simulink model "brain"  (Simulink 7.5)
settings: Solver=FixedStepDiscrete  StartTime=0.0  StopTime=inf  FixedStep=0.2  RelTol=1e-3
values from neighbouring files (symbols this model uses):
  Buoy1_Hue = 0.4    [brainconstants.m]    (also in brainconstants_David.m = 30)
  Buoy1_Saturation = 1.0    (= 1)    [brainconstants.m]    (also in brainconstants_David.m)
  Buoy1_Value = 0.45    [brainconstants.m]    (also in brainconstants_David.m)
  Buoy2_Hue = 0.0    (= 0)    [brainconstants.m]    (also in brainconstants_David.m = 80)
  Buoy2_Saturation = 1.0    (= 1)    [brainconstants.m]    (also in brainconstants_David.m)
  Buoy2_Value = 0.75    [brainconstants.m]    (also in brainconstants_David.m)
  Buoy_Max_Eccentricity = 0.7    [brainconstants.m]    (also in brainconstants_David.m = 1.2)
  Buoy_Max_Extent = 0.9    [brainconstants.m]    (also in brainconstants_David.m)
  Buoy_Min_Eccentricity = 0    [brainconstants.m]    (also in brainconstants_David.m)
  Buoy_Min_Extent = 0.7    [brainconstants.m]    (also in brainconstants_David.m = 0.1)
  Buoy_Strafe = 40    [brainconstants.m]    (also in brainconstants_David.m)
  Cam_Down_Strafe_XPos_Kd = 0.0    (= 0)    [brainconstants.m]    (also in brainconstants_David.m)
  Cam_Down_Strafe_XPos_Ki = 0.0    (= 0)    [brainconstants.m]    (also in brainconstants_David.m)
  Cam_Down_Strafe_XPos_Kp = -1.0    (= -1)    [brainconstants.m]    (also in brainconstants_David.m)
  Cam_Down_Yaw_XPos_Kd = 0.0    (= 0)    [brainconstants.m]    (also in brainconstants_David.m)
  Cam_Down_Yaw_XPos_Ki = 0.0    (= 0)    [brainconstants.m]    (also in brainconstants_David.m)
  Cam_Down_Yaw_XPos_Kp = 0.6    [brainconstants.m]    (also in brainconstants_David.m)
  Cam_Down_YPos_Kd = 0.0    (= 0)    [brainconstants.m]    (also in brainconstants_David.m)
  Cam_Down_YPos_Ki = 0.0    (= 0)    [brainconstants.m]    (also in brainconstants_David.m)
  Cam_Down_YPos_Kp = 0.75    [brainconstants.m]    (also in brainconstants_David.m)
  Cam_Forward_XPosition_Kd = 0.0    (= 0)    [brainconstants.m]    (also in brainconstants_David.m)
  Cam_Forward_XPosition_Ki = 0.0    (= 0)    [brainconstants.m]    (also in brainconstants_David.m)
  Cam_Forward_XPosition_Kp = 0.07    [brainconstants.m]    (also in brainconstants_David.m)
  Cam_Forward_YPosition_Kd = 0.0    (= 0)    [brainconstants.m]    (also in brainconstants_David.m)
  Cam_Forward_YPosition_Ki = 0.0    (= 0)    [brainconstants.m]    (also in brainconstants_David.m)
  Cam_Forward_YPosition_Kp = 0.8    [brainconstants.m]    (also in brainconstants_David.m)
  Depth_Kd = 0.0    (= 0)    [brainconstants.m]    (also in brainconstants_David.m)
  Depth_Ki = 0.0    (= 0)    [brainconstants.m]    (also in brainconstants_David.m)
  Depth_Kp = 75    [brainconstants.m]    (also in brainconstants_David.m)
  Heading_Forward_Velocity = 30    [brainconstants.m]    (also in brainconstants_David.m)
  Heading_Kd = 0.4    [brainconstants.m]    (also in brainconstants_David.m)
  Heading_Ki = 0.0    (= 0)    [brainconstants.m]    (also in brainconstants_David.m)
  Heading_Kp = 0.65    [brainconstants.m]    (also in brainconstants_David.m)
  Hedge_Hue = .4    (= 0.4)    [brainconstants.m]    (also in brainconstants_David.m)
  Hedge_Saturation = 1    [brainconstants.m]    (also in brainconstants_David.m)
  Hedge_Value = .75    (= 0.75)    [brainconstants.m]    (also in brainconstants_David.m)
  IMU_YawRate_Kd = 0.0    (= 0)    [brainconstants.m]    (also in brainconstants_David.m)
  IMU_YawRate_Ki = 0.0    (= 0)    [brainconstants.m]    (also in brainconstants_David.m)
  IMU_YawRate_Kp = 0.25    [brainconstants.m]    (also in brainconstants_David.m)
  IMU_YVel_Kd = 0.0    (= 0)    [brainconstants.m]    (also in brainconstants_David.m)
  IMU_YVel_Ki = 0.0    (= 0)    [brainconstants.m]    (also in brainconstants_David.m)
  IMU_YVel_Kp = 0.25    [brainconstants.m]    (also in brainconstants_David.m)
  Iter_Segment_Thresh = 60    [brainconstants.m]    (also in brainconstants_David.m)
  MissionPlan = [1 1 1 1 1 1 1 1 1 1 1 1 1 0 0 0 0 0 0 0]    [brainconstants.m]    (also in brainconstants_David.m)
  Track_Desired_Depth = 8    [brainconstants.m]    (also in brainconstants_David.m)
  Track_HueHigher = 0.75    [brainconstants.m]    (also in brainconstants_David.m)
  Track_HueLower = 0.4    [brainconstants.m]    (also in brainconstants_David.m)
  Track_Min_Eccentricity = 0.9    [brainconstants.m]    (also in brainconstants_David.m)
  Track_Saturation = 0.75    [brainconstants.m]    (also in brainconstants_David.m)
  Vision_Forward_Velocity = 15    [brainconstants.m]    (also in brainconstants_David.m)
undefined symbols (not defined in the file or in its folder): DiscIntNeverNeededParam, gray, Rec, SDTV, strel
libraries: vipconversions x32, simulink x26, vipgeotforms x9, vipstatistics x9, viptextngfix x7, vipmorphops x6, viptransforms x4, vipsnks x3, vipsrcs x1
(part 2 of 6)

== system brain/StateFlow Functions/StateFlowFunctions.GetDesiredDepth ==
  f : TriggerPort  TriggerType=function-call
      settings: CopyFcn=set_param(gcbh,'PreDeleteFcn','')  PreDeleteFcn=Stateflow.SLINSF.SimulinkMan.unsafePredeleteFcn
  Constant : Constant  Value=Track_Desired_Depth  OutDataType=fixdt(1, 16)  OutScaling=2^0  SampleTime=-1
  DesiredDepth : Outport
  wires:
  Constant/1 -> DesiredDepth/1

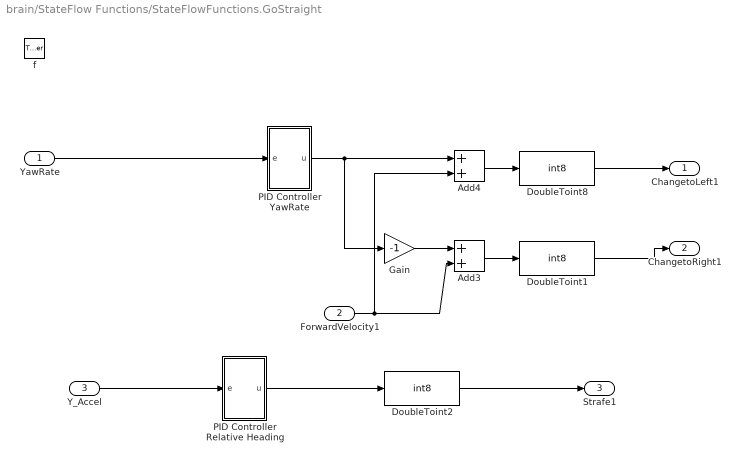
== system brain/StateFlow Functions/StateFlowFunctions.GoStraight ==
  YawRate : Inport
  ForwardVelocity1 : Inport  Port=2  OutDataType=fixdt(1, 16)  OutScaling=2^0
  Y_Accel : Inport  Port=3
  f : TriggerPort  TriggerType=function-call
      settings: CopyFcn=set_param(gcbh,'PreDeleteFcn','')  PreDeleteFcn=Stateflow.SLINSF.SimulinkMan.unsafePredeleteFcn
  Add3 : Sum  OutDataType=fixdt(1, 16)  OutScaling=2^-10
  Add4 : Sum  OutDataType=fixdt(1, 16)  OutScaling=2^-10
  DoubleToint1 : DataTypeConversion  OutDataTypeMode=int8  OutDataType=fixdt(1, 16)  OutScaling=2^0  OutDataTypeStr=int8  SaturateOnIntegerOverflow=on
  DoubleToint2 : DataTypeConversion  OutDataTypeMode=int8  OutDataType=fixdt(1, 16)  OutScaling=2^0  OutDataTypeStr=int8  SaturateOnIntegerOverflow=on
  DoubleToint8 : DataTypeConversion  OutDataTypeMode=int8  OutDataType=fixdt(1, 16)  OutScaling=2^0  OutDataTypeStr=int8  SaturateOnIntegerOverflow=on
  Gain : Gain  Gain=-1  ParameterDataType=fixdt(1, 16)  ParameterScaling=2^0  OutDataType=fixdt(1, 16)  OutScaling=2^0
  PID Controller Relative Heading : Subsystem  Description=PID
  PID Controller YawRate : Subsystem  Description=PID
  ChangetoLeft1 : Outport  OutDataType=fixdt(1, 16)  OutScaling=2^0
  ChangetoRight1 : Outport  Port=2  OutDataType=fixdt(1, 16)  OutScaling=2^0
  Strafe1 : Outport  Port=3  OutDataType=fixdt(1, 16)  OutScaling=2^0
  wires:
  PID Controller YawRate/1(u) -> Add4/1, Gain/1
  Add4/1 -> DoubleToint8/1
  Add3/1 -> DoubleToint1/1
  ForwardVelocity1/1 -> Add4/2, Add3/2
  YawRate/1 -> PID Controller YawRate/1(e)
  Gain/1 -> Add3/1
  DoubleToint8/1 -> ChangetoLeft1/1
  DoubleToint1/1 -> ChangetoRight1/1
  Y_Accel/1 -> PID Controller Relative Heading/1(e)
  PID Controller Relative Heading/1(u) -> DoubleToint2/1
  DoubleToint2/1 -> Strafe1/1

== system brain/StateFlow Functions/StateFlowFunctions.JumpHedge.ApproachHedge.GetArea ==
  BW : Inport  PortDimensions=[120 160]
  f : TriggerPort  TriggerType=function-call
      settings: CopyFcn=set_param(gcbh,'PreDeleteFcn','')  PreDeleteFcn=Stateflow.SLINSF.SimulinkMan.unsafePredeleteFcn
  Buoy Blob Analysis : vipstatistics/Blob Analysis  Tag=vipblks_row_conv  DialogController=vipDDGCreate  DialogControllerArgs=DataTag25  area=on  centroid=off  bBox=off  majorAxis=off  minorAxis=off  angle=off  eccentricity=off  equivDiameterSq=off  extent=off  perimeter=off  maxBlobs=Max_Num_Blobs  warnIfNumBlobsExceeded=off  isCount=off  useMinArea=on  minArea=Min_Blob_Size  useMaxArea=on  maxArea=Max_Blob_Size  excludeBorderBlob=off  outDT=double  isOutVarDim=off  isFill=on  fillValues=-1  conn=8  isLabel=off  outputMode=Binary point scaling  outputWordLength=32  outputFracLength=16  firstCoeffMode=Binary point scaling  firstCoeffWordLength=16  firstCoeffFracLength=14  secondCoeffMode=Binary point scaling  secondCoeffWordLength=32  secondCoeffFracLength=16  accumMode=Binary point scaling  accumWordLength=32  accumFracLength=0  prodOutputMode=Binary point scaling  prodOutputWordLength=32  prodOutputFracLength=16  roundingMode=Floor  overflowMode=off
  Dilation : vipmorphops/Dilation  nhoodsrc=Specify via dialog  strel=[1 1; 1 1]
  Embedded MATLAB Function : Stateflow chart  TreatAsAtomicUnit=on
  Erosion : vipmorphops/Erosion  nhoodsrc=Specify via dialog  strel=strel('square',4)
  Image Data Type Conversion : vipconversions/Image Data Type Conversion  outDT=boolean  isSigned=on  wordLen=16  numFracBits=0
  AreaBiggestBlob : Outport  OutDataType=fixdt(1, 16)  OutScaling=2^0
  wires:
  Buoy Blob Analysis/1 -> Embedded MATLAB Function/1(Area1)
  BW/1 -> Image Data Type Conversion/1  "BW"
  Dilation/1 -> Erosion/1
  Erosion/1 -> Buoy Blob Analysis/1, Embedded MATLAB Function/2(Image)
  Embedded MATLAB Function/1(BlobArea) -> AreaBiggestBlob/1
  Image Data Type Conversion/1 -> Dilation/1

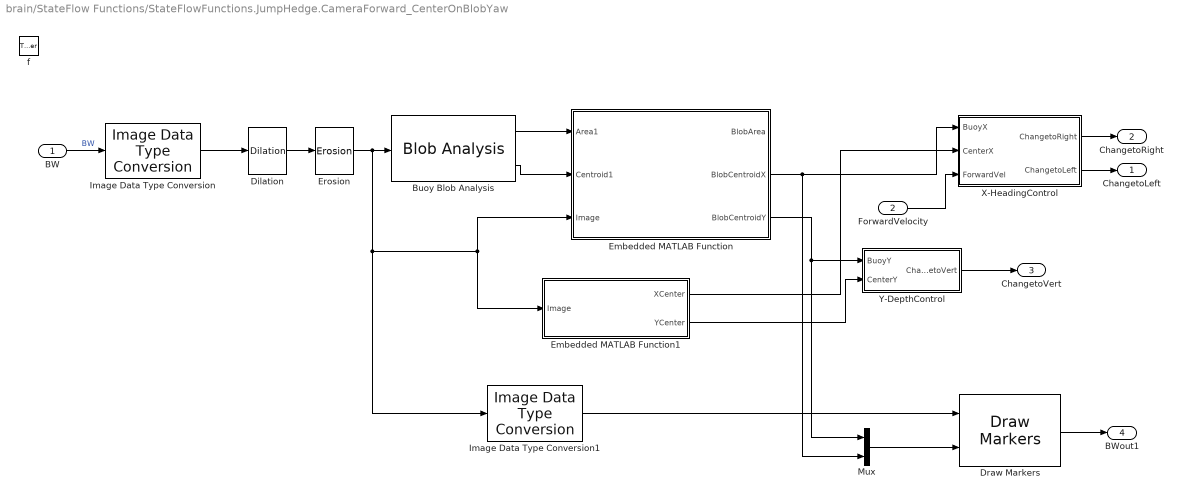
== system brain/StateFlow Functions/StateFlowFunctions.JumpHedge.CameraForward_CenterOnBlobYaw ==
  BW : Inport  PortDimensions=[120 160]
  ForwardVelocity : Inport  Port=2  PortDimensions=1
  f : TriggerPort  TriggerType=function-call
      settings: CopyFcn=set_param(gcbh,'PreDeleteFcn','')  PreDeleteFcn=Stateflow.SLINSF.SimulinkMan.unsafePredeleteFcn
  Buoy Blob Analysis : vipstatistics/Blob Analysis  Tag=vipblks_row_conv  DialogController=vipDDGCreate  DialogControllerArgs=DataTag26  area=on  centroid=on  bBox=off  majorAxis=off  minorAxis=off  angle=off  eccentricity=off  equivDiameterSq=off  extent=off  perimeter=off  maxBlobs=Max_Num_Blobs_Buoy  warnIfNumBlobsExceeded=off  isCount=off  useMinArea=on  minArea=Min_Blob_Size  useMaxArea=on  maxArea=Max_Blob_Size  excludeBorderBlob=off  outDT=double  isOutVarDim=off  isFill=on  fillValues=-1  conn=8  isLabel=off  outputMode=Binary point scaling  outputWordLength=32  outputFracLength=16  firstCoeffMode=Binary point scaling  firstCoeffWordLength=16  firstCoeffFracLength=14  secondCoeffMode=Binary point scaling  secondCoeffWordLength=32  secondCoeffFracLength=16  accumMode=Binary point scaling  accumWordLength=32  accumFracLength=0  prodOutputMode=Binary point scaling  prodOutputWordLength=32  prodOutputFracLength=16  roundingMode=Floor  overflowMode=off
  Dilation : vipmorphops/Dilation  nhoodsrc=Specify via dialog  strel=[1 1; 1 1]
  Draw Markers : viptextngfix/Draw Markers  DialogController=vipDDGCreate  DialogControllerArgs=DataTag27  shape=X-mark  size=7  fill=off  fillClrSource=Specify via dialog  display=User-specified value  intensity=200  color=.5  opacity=0.6  viewport=Entire image  antialiasing=off  inType=Obsolete  imagePorts=One multidimensional signal  prodOutputMode=Binary point scaling  prodOutputWordLength=32  prodOutputFracLength=14  memoryMode=Specify word length  memoryWordLength=16  memoryFracLength=15  roundingMode=Floor  overflowMode=off
  Embedded MATLAB Function : Stateflow chart  TreatAsAtomicUnit=on
  Embedded MATLAB Function1 : Stateflow chart  TreatAsAtomicUnit=on
  Erosion : vipmorphops/Erosion  nhoodsrc=Specify via dialog  strel=strel('square',4)
  Image Data Type Conversion : vipconversions/Image Data Type Conversion  outDT=boolean  isSigned=on  wordLen=16  numFracBits=0
  Image Data Type Conversion1 : vipconversions/Image Data Type Conversion  outDT=double  isSigned=on  wordLen=16  numFracBits=0
  Mux : Mux  Inputs=2
  X-HeadingControl : Subsystem
  Y-DepthControl : Subsystem
  ChangetoLeft : Outport  PortDimensions=1  OutDataType=fixdt(1, 16)  OutScaling=2^0
  ChangetoRight : Outport  Port=2  PortDimensions=1  OutDataType=fixdt(1, 16)  OutScaling=2^0
  ChangetoVert : Outport  Port=3  PortDimensions=1  OutDataType=fixdt(1, 16)  OutScaling=2^0
  BWout1 : Outport  Port=4  OutDataType=fixdt(1, 16)  OutScaling=2^0
  wires:
  X-HeadingControl/1(ChangetoRight) -> ChangetoRight/1
  X-HeadingControl/2(ChangetoLeft) -> ChangetoLeft/1
  Y-DepthControl/1(ChangetoVert) -> ChangetoVert/1
  Buoy Blob Analysis/1 -> Embedded MATLAB Function/1(Area1)
  Buoy Blob Analysis/2 -> Embedded MATLAB Function/2(Centroid1)
  Embedded MATLAB Function/2(BlobCentroidX) -> X-HeadingControl/1(BuoyX), Mux/2
  Embedded MATLAB Function/3(BlobCentroidY) -> Y-DepthControl/1(BuoyY), Mux/1
  BW/1 -> Image Data Type Conversion/1  "BW"
  Embedded MATLAB Function1/1(XCenter) -> X-HeadingControl/2(CenterX)
  Embedded MATLAB Function1/2(YCenter) -> Y-DepthControl/2(CenterY)
  Dilation/1 -> Erosion/1
  Erosion/1 -> Buoy Blob Analysis/1, Embedded MATLAB Function/3(Image), Embedded MATLAB Function1/1(Image), Image Data Type Conversion1/1
  ForwardVelocity/1 -> X-HeadingControl/3(ForwardVel)
  Image Data Type Conversion/1 -> Dilation/1
  Mux/1 -> Draw Markers/2
  Image Data Type Conversion1/1 -> Draw Markers/1
  Draw Markers/1 -> BWout1/1

== system brain/StateFlow Functions/StateFlowFunctions.JumpHedge.GetAxisRatio ==
  BW : Inport  PortDimensions=[120 160]
  f : TriggerPort  TriggerType=function-call
      settings: CopyFcn=set_param(gcbh,'PreDeleteFcn','')  PreDeleteFcn=Stateflow.SLINSF.SimulinkMan.unsafePredeleteFcn
  Blob Analysis : vipstatistics/Blob Analysis  Tag=vipblks_row_conv  DialogController=vipDDGCreate  DialogControllerArgs=DataTag28  area=on  centroid=off  bBox=on  majorAxis=off  minorAxis=off  angle=off  eccentricity=off  equivDiameterSq=off  extent=off  perimeter=off  maxBlobs=10  warnIfNumBlobsExceeded=on  isCount=off  useMinArea=off  minArea=0  useMaxArea=off  maxArea=intmax('uint32')  excludeBorderBlob=off  outDT=double  isOutVarDim=off  isFill=on  fillValues=-1  conn=8  isLabel=off  outputMode=Binary point scaling  outputWordLength=32  outputFracLength=16  firstCoeffMode=Binary point scaling  firstCoeffWordLength=16  firstCoeffFracLength=14  secondCoeffMode=Binary point scaling  secondCoeffWordLength=32  secondCoeffFracLength=16  accumMode=Binary point scaling  accumWordLength=32  accumFracLength=0  prodOutputMode=Binary point scaling  prodOutputWordLength=32  prodOutputFracLength=16  roundingMode=Floor  overflowMode=off
  Embedded MATLAB Function : Stateflow chart  TreatAsAtomicUnit=on
  Image Data Type Conversion : vipconversions/Image Data Type Conversion  outDT=boolean  isSigned=on  wordLen=16  numFracBits=0
  AxisRatio : Outport
  wires:
  BW/1 -> Image Data Type Conversion/1
  Blob Analysis/1 -> Embedded MATLAB Function/1(Area1)
  Blob Analysis/2 -> Embedded MATLAB Function/2(BBox)
  Embedded MATLAB Function/2(AxisRatio) -> AxisRatio/1
  Image Data Type Conversion/1 -> Blob Analysis/1, Embedded MATLAB Function/3(Image)

== system brain/StateFlow Functions/StateFlowFunctions.JumpHedge.GetForwardVelocity ==
  f : TriggerPort  TriggerType=function-call
      settings: CopyFcn=set_param(gcbh,'PreDeleteFcn','')  PreDeleteFcn=Stateflow.SLINSF.SimulinkMan.unsafePredeleteFcn
  Heading Forward Velocity : Constant  Value=Vision_Forward_Velocity  OutDataType=fixdt(1, 16)  OutScaling=2^0  SampleTime=-1
  ForwardVel : Outport
  wires:
  Heading Forward Velocity/1 -> ForwardVel/1

== system brain/StateFlow Functions/StateFlowFunctions.JumpHedge.IndividualSegmentation ==
  LabMatrix : Inport  PortDimensions=[120 160]
  Ref_Colors : Inport  Port=2  PortDimensions=[50 3]
  Num_Colors : Inport  Port=3  PortDimensions=1
  B_Hue : Inport  Port=4
  B_Sat : Inport  Port=5
  B_Value : Inport  Port=6
  f : TriggerPort  TriggerType=function-call
      settings: CopyFcn=set_param(gcbh,'PreDeleteFcn','')  PreDeleteFcn=Stateflow.SLINSF.SimulinkMan.unsafePredeleteFcn
  Threshold The Image : Subsystem
  BW : Outport  PortDimensions=[120 160]  OutDataType=fixdt(1, 16)  OutScaling=2^0
  wires:
  LabMatrix/1 -> Threshold The Image/1(LabelMatrix)
  Ref_Colors/1 -> Threshold The Image/2(ref_colors)
  Num_Colors/1 -> Threshold The Image/3(num_colors)
  B_Hue/1 -> Threshold The Image/4(H_Hue)
  B_Sat/1 -> Threshold The Image/5(H_Sat)
  B_Value/1 -> Threshold The Image/6(H_Value)
  Threshold The Image/1(BW) -> BW/1

== system brain/StateFlow Functions/StateFlowFunctions.JumpHedge.IterativeSegmentation ==
  H : Inport  PortDimensions=[120 160]
  S : Inport  Port=2  PortDimensions=[120 160]
  V : Inport  Port=3  PortDimensions=[120 160]
  f : TriggerPort  TriggerType=function-call
      settings: CopyFcn=set_param(gcbh,'PreDeleteFcn','')  PreDeleteFcn=Stateflow.SLINSF.SimulinkMan.unsafePredeleteFcn
  Color Space  Conversion : vipconversions/Color Space  Conversion  conversion=Obsolete  conversionActive=HSV to R'G'B'  wp_str=D50  rec=Rec. 601 (SDTV)  sys=1125/60/2:1  imagePorts=Separate color signals
  Color Space  Conversion1 : vipconversions/Color Space  Conversion  conversion=Obsolete  conversionActive=sR'G'B' to L*a*b*  wp_str=D50  rec=Rec. 601 (SDTV)  sys=1125/60/2:1  imagePorts=Separate color signals
  Low Pass Filter : Subsystem
  Segmentation : Subsystem
  LabelMatrix : Outport  PortDimensions=[120 160]
  num_colors : Outport  Port=2
  Ref_Colors : Outport  Port=3
  wires:
  Color Space  Conversion/1 -> Low Pass Filter/1(R)
  Color Space  Conversion/2 -> Low Pass Filter/2(G)
  Color Space  Conversion/3 -> Low Pass Filter/3(B)
  Color Space  Conversion1/1 -> Segmentation/1(L)
  Color Space  Conversion1/2 -> Segmentation/2(a)
  Color Space  Conversion1/3 -> Segmentation/3(b)
  Low Pass Filter/1(R') -> Color Space  Conversion1/1
  Low Pass Filter/2(G') -> Color Space  Conversion1/2
  Low Pass Filter/3(B') -> Color Space  Conversion1/3
  H/1 -> Color Space  Conversion/1
  S/1 -> Color Space  Conversion/2
  V/1 -> Color Space  Conversion/3
  Segmentation/1(LabelMatrix) -> LabelMatrix/1
  Segmentation/2(num_colors) -> num_colors/1
  Segmentation/3(ref_colors) -> Ref_Colors/1

== system brain/StateFlow Functions/StateFlowFunctions.JumpHedge.RecognizeHedge.GetHedgeValues ==
  f : TriggerPort  TriggerType=function-call
      settings: CopyFcn=set_param(gcbh,'PreDeleteFcn','')  PreDeleteFcn=Stateflow.SLINSF.SimulinkMan.unsafePredeleteFcn
  Hedge Hue : Constant  Value=Hedge_Hue  OutDataType=fixdt(1, 16)  OutScaling=2^0  SampleTime=-1
  Hedge Saturation : Constant  Value=Hedge_Saturation  OutDataType=fixdt(1, 16)  OutScaling=2^0  SampleTime=-1
  Hedge Value : Constant  Value=Hedge_Value  OutDataType=fixdt(1, 16)  OutScaling=2^0  SampleTime=-1
  H_hue : Outport
  H_sat : Outport  Port=2
  H_val : Outport  Port=3
  wires:
  Hedge Hue/1 -> H_hue/1
  Hedge Saturation/1 -> H_sat/1
  Hedge Value/1 -> H_val/1

== system brain/StateFlow Functions/StateFlowFunctions.JumpHedge.RecognizeHedge.LookForHedge ==
  BW : Inport  PortDimensions=[120 160]
  f : TriggerPort  TriggerType=function-call
      settings: CopyFcn=set_param(gcbh,'PreDeleteFcn','')  PreDeleteFcn=Stateflow.SLINSF.SimulinkMan.unsafePredeleteFcn
  Are 3 Lines Present : Stateflow chart  TreatAsAtomicUnit=on
  Draw Shapes : viptextngfix/Draw Shapes  DialogController=vipDDGCreate  DialogControllerArgs=DataTag32  shape=Lines  fill=off  fillClrSource=Specify via dialog  display=User-specified value  intensity=200  color=.8  opacity=0.6  viewport=Entire image  antialiasing=off  inType=Obsolete  imagePorts=One multidimensional signal  prodOutputMode=Binary point scaling  prodOutputWordLength=32  prodOutputFracLength=14  memoryMode=Specify word length  memoryWordLength=16  memoryFracLength=15  roundingMode=Floor  overflowMode=off
  Erosion : vipmorphops/Erosion  nhoodsrc=Specify via dialog  strel=[1 1 1;1 1 1]
  Hough Lines : viptransforms/Hough Lines  DialogController=vipDDGCreate  DialogControllerArgs=DataTag33  sineCompMethod=Trigonometric function  thetaRes=pi/180  firstCoeffMode=Specify word length  firstCoeffWordLength=16  firstCoeffFracLength=15  prodOutputMode=Binary point scaling  prodOutputWordLength=32  prodOutputFracLength=16  roundingMode=Nearest  overflowMode=on
  Hough Transform : viptransforms/Hough Transform  DialogController=vipDDGCreate  DialogControllerArgs=DataTag34  theta_res=pi/180  rho_res=1  out_theta_rho=on  outdtmode=double  firstCoeffMode=Binary point scaling  firstCoeffWordLength=16  firstCoeffFracLength=14  secondCoeffMode=Binary point scaling  secondCoeffWordLength=32  secondCoeffFracLength=16  outputMode=Binary point scaling  outputWordLength=16  outputFracLength=0  accumMode=Binary point scaling  accumWordLength=32  accumFracLength=20  prodOutputMode=Binary point scaling  prodOutputWordLength=32  prodOutputFracLength=20  memoryMode=Binary point scaling  memoryWordLength=32  memoryFracLength=16  roundingMode=Nearest  overflowMode=on
  Image Data Type Conversion : vipconversions/Image Data Type Conversion  outDT=boolean  isSigned=on  wordLen=16  numFracBits=0
  Image1 : Outport
  BWout1 : Outport  Port=2  PortDimensions=[120 160]
  wires:
  BW/1 -> Image Data Type Conversion/1, Hough Lines/3, Draw Shapes/1
  Hough Transform/1 -> Are 3 Lines Present/1(HoughTable)
  Hough Transform/2 -> Are 3 Lines Present/2(Theta)
  Hough Transform/3 -> Are 3 Lines Present/3(Rho)
  Are 3 Lines Present/1(Image) -> Image1/1
  Are 3 Lines Present/2(T) -> Hough Lines/1
  Are 3 Lines Present/3(R) -> Hough Lines/2
  Hough Lines/1 -> Draw Shapes/2
  Draw Shapes/1 -> BWout1/1
  Erosion/1 -> Hough Transform/1
  Image Data Type Conversion/1 -> Erosion/1

== system brain/StateFlow Functions/StateFlowFunctions.JumpHedge.ShowSegmentedImage ==
  LabMatrix : Inport  PortDimensions=[120 160]
  Ref_Colors : Inport  Port=2  PortDimensions=[50 3]
  f : TriggerPort  TriggerType=function-call
      settings: CopyFcn=set_param(gcbh,'PreDeleteFcn','')  PreDeleteFcn=Stateflow.SLINSF.SimulinkMan.unsafePredeleteFcn
  Color Space  Conversion : vipconversions/Color Space  Conversion  conversion=Obsolete  conversionActive=L*a*b* to sR'G'B'  wp_str=D50  rec=Rec. 601 (SDTV)  sys=1125/60/2:1  imagePorts=Separate color signals
  Embedded MATLAB Function : Stateflow chart  TreatAsAtomicUnit=on
  Embedded MATLAB Function1 : Stateflow chart  TreatAsAtomicUnit=on
  RGBout : Outport  PortDimensions=[120 160 3]  OutDataType=fixdt(1, 16)  OutScaling=2^0
  wires:
  LabMatrix/1 -> Embedded MATLAB Function/1(LabMatrix)
  Ref_Colors/1 -> Embedded MATLAB Function/2(Ref_Colors)
  Embedded MATLAB Function/1(L) -> Color Space  Conversion/1
  Embedded MATLAB Function/2(a) -> Color Space  Conversion/2
  Embedded MATLAB Function/3(b) -> Color Space  Conversion/3
  Color Space  Conversion/1 -> Embedded MATLAB Function1/1(R)
  Color Space  Conversion/2 -> Embedded MATLAB Function1/2(G)
  Color Space  Conversion/3 -> Embedded MATLAB Function1/3(B)
  Embedded MATLAB Function1/1(RGB) -> RGBout/1

== system brain/StateFlow Functions/StateFlowFunctions.LocatePinger.GetPingerHeading.GetHeadings ==
  f : TriggerPort  TriggerType=function-call
      settings: CopyFcn=set_param(gcbh,'PreDeleteFcn','')  PreDeleteFcn=Stateflow.SLINSF.SimulinkMan.unsafePredeleteFcn
  Heading11 : Outport
  Heading22 : Outport  Port=2

== system brain/StateFlow Functions/StateFlowFunctions.MaintainDepth ==
  note: Error
  CurrentDepth1 : Inport  DataType=single  OutDataType=fixdt(1, 16)  OutScaling=2^0  OutDataTypeStr=single
  DesiredDepth1 : Inport  Port=2  DataType=single  OutDataType=fixdt(1, 16)  OutScaling=2^0  OutDataTypeStr=single
  f : TriggerPort  TriggerType=function-call
      settings: CopyFcn=set_param(gcbh,'PreDeleteFcn','')  PreDeleteFcn=Stateflow.SLINSF.SimulinkMan.unsafePredeleteFcn
  Add : Sum  Inputs=+-  OutDataTypeMode=double  OutDataType=fixdt(1, 16)  OutScaling=2^-10  OutDataTypeStr=double
  Double To Int8 : DataTypeConversion  OutDataTypeMode=int8  OutDataType=fixdt(1, 16)  OutScaling=2^0  OutDataTypeStr=int8  SaturateOnIntegerOverflow=on
  PID Controller Depth S3 : Subsystem  Description=PID
  ChangetoVertical : Outport  DataType=int8  OutDataType=fixdt(1, 16)  OutScaling=2^0  OutDataTypeStr=int8
  wires:
  DesiredDepth1/1 -> Add/1
  CurrentDepth1/1 -> Add/2
  Double To Int8/1 -> ChangetoVertical/1
  PID Controller Depth S3/1(u) -> Double To Int8/1
  Add/1 -> PID Controller Depth S3/1(e)

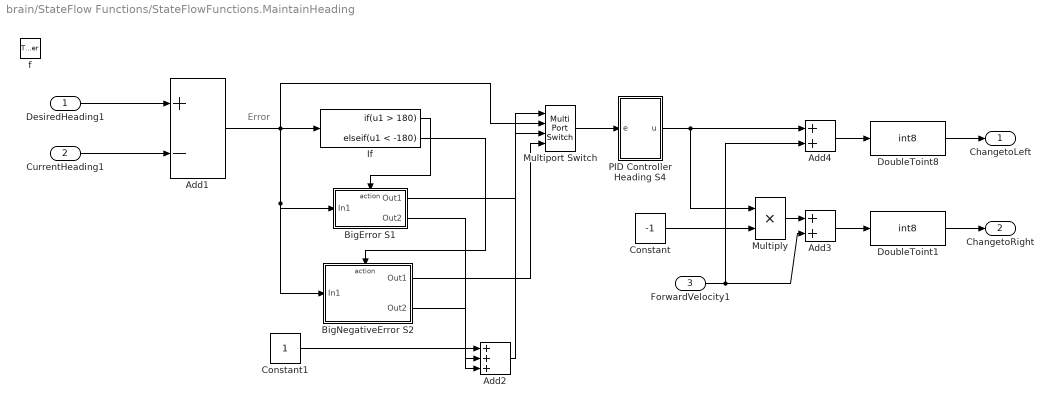
== system brain/StateFlow Functions/StateFlowFunctions.MaintainHeading ==
  note: Error
  DesiredHeading1 : Inport  PortDimensions=1  OutDataType=fixdt(1, 16)  OutScaling=2^0
  CurrentHeading1 : Inport  Port=2  PortDimensions=1  OutDataType=fixdt(1, 16)  OutScaling=2^0
  ForwardVelocity1 : Inport  Port=3  OutDataType=fixdt(1, 16)  OutScaling=2^0
  f : TriggerPort  TriggerType=function-call
      settings: CopyFcn=set_param(gcbh,'PreDeleteFcn','')  PreDeleteFcn=Stateflow.SLINSF.SimulinkMan.unsafePredeleteFcn
  Add1 : Sum  Inputs=+-  AccumDataTypeStr=double  OutDataType=fixdt(1, 16)  OutScaling=2^-10
  Add2 : Sum  Inputs=+++  OutDataType=fixdt(1, 16)  OutScaling=2^-10
  Add3 : Sum  OutDataType=fixdt(1, 16)  OutScaling=2^-10
  Add4 : Sum  OutDataType=fixdt(1, 16)  OutScaling=2^-10
  BigError S1 : Subsystem  TreatAsAtomicUnit=on
  BigNegativeError S2 : Subsystem  TreatAsAtomicUnit=on
  Constant : Constant  Value=-1  OutDataTypeMode=int8  OutDataType=fixdt(1, 16)  OutScaling=2^0  OutDataTypeStr=int8  SampleTime=-1
  Constant1 : Constant  OutDataType=fixdt(1, 16)  OutScaling=2^0  SampleTime=-1
  DoubleToint1 : DataTypeConversion  OutDataTypeMode=int8  OutDataType=fixdt(1, 16)  OutScaling=2^0  OutDataTypeStr=int8  SaturateOnIntegerOverflow=on
  DoubleToint8 : DataTypeConversion  OutDataTypeMode=int8  OutDataType=fixdt(1, 16)  OutScaling=2^0  OutDataTypeStr=int8  SaturateOnIntegerOverflow=on
  If : If  IfExpression=u1 > 180  ElseIfExpressions=u1 < -180  ShowElse=off
  Multiply : Product  Inputs=**  OutDataTypeMode=int8  OutDataType=fixdt(1, 16)  OutScaling=2^-10  OutDataTypeStr=int8
  Multiport Switch : MultiPortSwitch  zeroidx=off  OutDataType=fixdt(1, 16)  OutScaling=2^0
  PID Controller Heading S4 : Subsystem  Description=PID
  ChangetoLeft : Outport  OutDataType=fixdt(1, 16)  OutScaling=2^0
  ChangetoRight : Outport  Port=2  OutDataType=fixdt(1, 16)  OutScaling=2^0
  wires:
  PID Controller Heading S4/1(u) -> Multiply/1, Add4/1
  DoubleToint8/1 -> ChangetoLeft/1
  Add4/1 -> DoubleToint8/1
  DoubleToint1/1 -> ChangetoRight/1
  Add3/1 -> DoubleToint1/1
  ForwardVelocity1/1 -> Add4/2, Add3/2
  Multiply/1 -> Add3/1
  CurrentHeading1/1 -> Add1/2
  Add2/1 -> Multiport Switch/1
  BigNegativeError S2/2(Out2) -> Add2/3
  BigError S1/2(Out2) -> Add2/2
  Constant1/1 -> Add2/1
  Multiport Switch/1 -> PID Controller Heading S4/1(e)
  BigNegativeError S2/1(Out1) -> Multiport Switch/4
  BigError S1/1(Out1) -> Multiport Switch/3
  If/2 -> BigNegativeError S2/Action
  If/1 -> BigError S1/Action
  Add1/1 -> Multiport Switch/2, If/1, BigNegativeError S2/1(In1), BigError S1/1(In1)
  Constant/1 -> Multiply/2
  DesiredHeading1/1 -> Add1/1

== system brain/StateFlow Functions/StateFlowFunctions.ValidationGate.GetValidationGateForwardVelocity ==
  f : TriggerPort  TriggerType=function-call
      settings: CopyFcn=set_param(gcbh,'PreDeleteFcn','')  PreDeleteFcn=Stateflow.SLINSF.SimulinkMan.unsafePredeleteFcn
  Heading Forward Velocity : Constant  Value=Heading_Forward_Velocity  OutDataType=fixdt(1, 16)  OutScaling=2^0  SampleTime=-1
  ForwardVel : Outport
  wires:
  Heading Forward Velocity/1 -> ForwardVel/1

== system brain/StateFlow Functions/StateFlowFunctions.ValidationGate.LookforTrack ==
  H : Inport  PortDimensions=[120 160]  OutDataType=fixdt(1, 16)  OutScaling=2^0
  S : Inport  Port=2  PortDimensions=[120 160]  OutDataType=fixdt(1, 16)  OutScaling=2^0
  f : TriggerPort  TriggerType=function-call
      settings: CopyFcn=set_param(gcbh,'PreDeleteFcn','')  PreDeleteFcn=Stateflow.SLINSF.SimulinkMan.unsafePredeleteFcn
  LookforTrack : Subsystem
  Image : Outport  OutDataType=fixdt(1, 16)  OutScaling=2^0
  BWout1 : Outport  Port=2  OutDataType=fixdt(1, 16)  OutScaling=2^0
  wires:
  H/1 -> LookforTrack/1(H)
  S/1 -> LookforTrack/2(S)
  LookforTrack/1(BWout) -> BWout1/1
  LookforTrack/2(Image) -> Image/1

== system brain/StateFlow Functions/StateManagement.Running.Autonomous.Perform ==
  State1 : Inport
  f : TriggerPort  TriggerType=function-call
      settings: CopyFcn=set_param(gcbh,'PreDeleteFcn','')  PreDeleteFcn=Stateflow.SLINSF.SimulinkMan.unsafePredeleteFcn
  Checking to see if state will be performed : Stateflow chart  TreatAsAtomicUnit=on
  Mission Plan : Constant  Value=MissionPlan  OutDataType=fixdt(1, 16)  OutScaling=2^0  SampleTime=-1
  Done1 : Outport
  wires:
  State1/1 -> Checking to see if state will be performed/1(State1)
  Mission Plan/1 -> Checking to see if state will be performed/2(MissionPlan)
  Checking to see if state will be performed/1(Done1) -> Done1/1

== system brain/StateFlow Functions/StateFlowFunctions.Buoys.ApproachBuoys.ApproachFirstBuoy.WhichBuoysToApproach/FirstBuoy Info ==
  Color Space  Conversion : vipconversions/Color Space  Conversion  conversion=Obsolete  conversionActive=HSV to R'G'B'  wp_str=D65  rec=Rec. 601 (SDTV)  sys=1125/60/2:1  imagePorts=Separate color signals
  Color Space  Conversion1 : vipconversions/Color Space  Conversion  conversion=Obsolete  conversionActive=sR'G'B' to L*a*b*  wp_str=D50  rec=Rec. 601 (SDTV)  sys=1125/60/2:1  imagePorts=Separate color signals
  Constant : Constant  Value=Buoy1_Hue  OutDataType=fixdt(1, 16)  OutScaling=2^0  SampleTime=-1
  Constant1 : Constant  Value=Buoy1_Value  OutDataType=fixdt(1, 16)  OutScaling=2^0  SampleTime=-1
  Constant2 : Constant  Value=Buoy1_Saturation  OutDataType=fixdt(1, 16)  OutScaling=2^0  SampleTime=-1
  Out1 : Outport
  Out2 : Outport  Port=2
  Out3 : Outport  Port=3
  wires:
  Color Space  Conversion/1 -> Color Space  Conversion1/1
  Color Space  Conversion/2 -> Color Space  Conversion1/2
  Color Space  Conversion/3 -> Color Space  Conversion1/3
  Constant/1 -> Color Space  Conversion/1
  Constant2/1 -> Color Space  Conversion/2
  Constant1/1 -> Color Space  Conversion/3
  Color Space  Conversion1/1 -> Out1/1
  Color Space  Conversion1/2 -> Out2/1
  Color Space  Conversion1/3 -> Out3/1

== system brain/StateFlow Functions/StateFlowFunctions.Buoys.ApproachBuoys.ApproachFirstBuoy.WhichBuoysToApproach/Second Buoy Info ==
  Color Space  Conversion : vipconversions/Color Space  Conversion  conversion=Obsolete  conversionActive=HSV to R'G'B'  wp_str=D65  rec=Rec. 601 (SDTV)  sys=1125/60/2:1  imagePorts=Separate color signals
  Color Space  Conversion1 : vipconversions/Color Space  Conversion  conversion=Obsolete  conversionActive=sR'G'B' to L*a*b*  wp_str=D50  rec=Rec. 601 (SDTV)  sys=1125/60/2:1  imagePorts=Separate color signals
  Constant : Constant  Value=Buoy2_Hue  OutDataType=fixdt(1, 16)  OutScaling=2^0  SampleTime=-1
  Constant1 : Constant  Value=Buoy2_Value  OutDataType=fixdt(1, 16)  OutScaling=2^0  SampleTime=-1
  Constant2 : Constant  Value=Buoy2_Saturation  OutDataType=fixdt(1, 16)  OutScaling=2^0  SampleTime=-1
  Out1 : Outport
  Out2 : Outport  Port=2
  Out3 : Outport  Port=3
  wires:
  Color Space  Conversion/1 -> Color Space  Conversion1/1
  Color Space  Conversion/2 -> Color Space  Conversion1/2
  Color Space  Conversion/3 -> Color Space  Conversion1/3
  Constant/1 -> Color Space  Conversion/1
  Constant2/1 -> Color Space  Conversion/2
  Constant1/1 -> Color Space  Conversion/3
  Color Space  Conversion1/1 -> Out1/1
  Color Space  Conversion1/2 -> Out2/1
  Color Space  Conversion1/3 -> Out3/1

== system brain/StateFlow Functions/StateFlowFunctions.Buoys.ApproachBuoys.Buoy/Threshold The Image ==
  LabelMatrix : Inport
  ref_colors : Inport  Port=2
  num_colors : Inport  Port=3
  B_Hue : Inport  Port=4
  B_Sat : Inport  Port=5
  B_Value : Inport  Port=6
  Choose Closest Color : Stateflow chart  TreatAsAtomicUnit=on
  Get Desired Color : Subsystem
  Relational Operator : RelationalOperator  Operator===  LogicOutDataTypeMode=boolean  LogicDataType=fixdt(0, 8)  OutDataTypeStr=boolean
  BW : Outport
  wires:
  Relational Operator/1 -> BW/1  "BW"
  ref_colors/1 -> Choose Closest Color/1(ref_colors)
  num_colors/1 -> Choose Closest Color/2(num_colors)
  Get Desired Color/1(L) -> Choose Closest Color/3(L)
  Get Desired Color/2(a) -> Choose Closest Color/4(a)
  Get Desired Color/3(b) -> Choose Closest Color/5(b)
  LabelMatrix/1 -> Relational Operator/1
  Choose Closest Color/1(index) -> Relational Operator/2
  B_Hue/1 -> Get Desired Color/1(B_Hue)
  B_Sat/1 -> Get Desired Color/2(B_Sat)
  B_Value/1 -> Get Desired Color/3(B_Value)

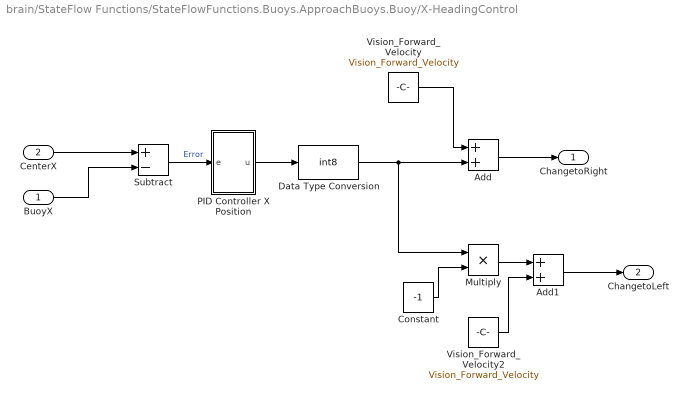
== system brain/StateFlow Functions/StateFlowFunctions.Buoys.ApproachBuoys.Buoy/X-HeadingControl ==
  BuoyX : Inport  OutDataType=fixdt(1, 16)  OutScaling=2^0
  CenterX : Inport  Port=2  OutDataType=fixdt(1, 16)  OutScaling=2^0
  Add : Sum  OutDataType=fixdt(1, 16)  OutScaling=2^-10
  Add1 : Sum  OutDataType=fixdt(1, 16)  OutScaling=2^-10
  Constant : Constant  Value=-1  OutDataType=fixdt(1, 16)  OutScaling=2^0  SampleTime=-1
  Data Type Conversion : DataTypeConversion  OutDataTypeMode=int8  OutDataType=fixdt(1, 16)  OutScaling=2^0  OutDataTypeStr=int8  SaturateOnIntegerOverflow=on
  Multiply : Product  Inputs=**  OutDataType=fixdt(1, 16)  OutScaling=2^-10
  PID Controller X Position : Subsystem  Description=PID
  Subtract : Sum  Inputs=+-  OutDataTypeMode=double  OutDataType=fixdt(1, 16)  OutScaling=2^-10  OutDataTypeStr=double
  Vision_Forward_Velocity : Constant  Value=Vision_Forward_Velocity  OutDataType=fixdt(1, 16)  OutScaling=2^0  SampleTime=-1
  Vision_Forward_Velocity2 : Constant  Value=Vision_Forward_Velocity  OutDataType=fixdt(1, 16)  OutScaling=2^0  SampleTime=-1
  ChangetoRight : Outport  OutDataType=fixdt(1, 16)  OutScaling=2^0
  ChangetoLeft : Outport  Port=2  OutDataType=fixdt(1, 16)  OutScaling=2^0
  wires:
  CenterX/1 -> Subtract/1
  BuoyX/1 -> Subtract/2
  Subtract/1 -> PID Controller X Position/1(e)  "Error"
  PID Controller X Position/1(u) -> Data Type Conversion/1
  Constant/1 -> Multiply/2
  Data Type Conversion/1 -> Multiply/1, Add/2
  Vision_Forward_Velocity/1 -> Add/1
  Add/1 -> ChangetoRight/1
  Multiply/1 -> Add1/1
  Vision_Forward_Velocity2/1 -> Add1/2
  Add1/1 -> ChangetoLeft/1

== system brain/StateFlow Functions/StateFlowFunctions.Buoys.ApproachBuoys.Buoy/Y-DepthControl ==
  BuoyY : Inport  OutDataType=fixdt(1, 16)  OutScaling=2^0
  CenterY : Inport  Port=2  OutDataType=fixdt(1, 16)  OutScaling=2^0
  Data Type Conversion : DataTypeConversion  OutDataTypeMode=int8  OutDataType=fixdt(1, 16)  OutScaling=2^0  OutDataTypeStr=int8  SaturateOnIntegerOverflow=on
  PID Controller Y Position : Subsystem  Description=PID
  Subtract : Sum  Inputs=-+  OutDataTypeMode=double  OutDataType=fixdt(1, 16)  OutScaling=2^-10  OutDataTypeStr=double
  ChangetoVert : Outport  OutDataType=fixdt(1, 16)  OutScaling=2^0
  wires:
  CenterY/1 -> Subtract/1
  BuoyY/1 -> Subtract/2
  Subtract/1 -> PID Controller Y Position/1(e)  "Error"
  PID Controller Y Position/1(u) -> Data Type Conversion/1
  Data Type Conversion/1 -> ChangetoVert/1

== system brain/StateFlow Functions/StateFlowFunctions.Buoys.ApproachBuoys.FindSecondBuoy.SecondBuoy/Threshold The Image ==
  LabelMatrix : Inport
  ref_colors : Inport  Port=2
  num_colors : Inport  Port=3
  B_Hue : Inport  Port=4
  B_Sat : Inport  Port=5
  B_Value : Inport  Port=6
  Choose Closest Color : Stateflow chart  TreatAsAtomicUnit=on
  Get Desired Color : Subsystem
  Relational Operator : RelationalOperator  Operator===  LogicOutDataTypeMode=boolean  LogicDataType=fixdt(0, 8)  OutDataTypeStr=boolean
  BW : Outport
  wires:
  Relational Operator/1 -> BW/1  "BW"
  ref_colors/1 -> Choose Closest Color/1(ref_colors)
  num_colors/1 -> Choose Closest Color/2(num_colors)
  Get Desired Color/1(L) -> Choose Closest Color/3(L)
  Get Desired Color/2(a) -> Choose Closest Color/4(a)
  Get Desired Color/3(b) -> Choose Closest Color/5(b)
  LabelMatrix/1 -> Relational Operator/1
  Choose Closest Color/1(index) -> Relational Operator/2
  B_Hue/1 -> Get Desired Color/1(B_Hue)
  B_Sat/1 -> Get Desired Color/2(B_Sat)
  B_Value/1 -> Get Desired Color/3(B_Value)

== system brain/StateFlow Functions/StateFlowFunctions.Buoys.IterativeSegmentation/Low Pass Filter ==
  R : Inport
  G : Inport  Port=2
  B : Inport  Port=3
  Low Pass Filter : Stateflow chart  TreatAsAtomicUnit=on
  Low Pass Filter1 : Stateflow chart  TreatAsAtomicUnit=on
  Low Pass Filter2 : Stateflow chart  TreatAsAtomicUnit=on
  R' : Outport
  G' : Outport  Port=2
  B' : Outport  Port=3
  wires:
  R/1 -> Low Pass Filter/1(I)
  G/1 -> Low Pass Filter1/1(I)
  B/1 -> Low Pass Filter2/1(I)
  Low Pass Filter1/1(Iout) -> G'/1
  Low Pass Filter2/1(Iout) -> B'/1
  Low Pass Filter/1(Iout) -> R'/1

== system brain/StateFlow Functions/StateFlowFunctions.Buoys.IterativeSegmentation/Segmentation ==
  L : Inport
  a : Inport  Port=2
  b : Inport  Port=3
  Dist_Thresh : Constant  Value=Iter_Segment_Thresh  OutDataType=fixdt(1, 16)  OutScaling=2^0  SampleTime=-1
  LabSegmentation : Stateflow chart  TreatAsAtomicUnit=on
  Reference Color Selection : Stateflow chart  TreatAsAtomicUnit=on
  Resize : Subsystem
  LabelMatrix : Outport
  num_colors : Outport  Port=2
  ref_colors : Outport  Port=3
  wires:
  L/1 -> Resize/1(In1), LabSegmentation/1(L)
  a/1 -> Resize/2(In2), LabSegmentation/2(a)
  b/1 -> Resize/3(In3), LabSegmentation/3(b)
  Resize/1(Out1) -> Reference Color Selection/1(L)
  Resize/2(Out2) -> Reference Color Selection/2(a)
  Resize/3(Out3) -> Reference Color Selection/3(b)
  Reference Color Selection/1(ref_colors) -> LabSegmentation/4(ref_colors), ref_colors/1
  Reference Color Selection/2(num_colors) -> LabSegmentation/5(num_colors), num_colors/1
  LabSegmentation/1(LabelMatrix) -> LabelMatrix/1
  Dist_Thresh/1 -> Reference Color Selection/4(Dist_Thresh)

== system brain/StateFlow Functions/StateFlowFunctions.FollowOnePath.OnePath.AlignWithPath.Align/PID Controller Relative Heading ==
  e : Inport
  CamDownStrafe-X Derivative Gain : Gain  Gain=Cam_Down_Strafe_XPos_Kd  ParameterDataType=fixdt(1, 16)  ParameterScaling=2^0  OutDataType=fixdt(1, 16)  OutScaling=2^0
  CamDownStrafe-X Integral Gain : Gain  Gain=Cam_Down_Strafe_XPos_Ki  ParameterDataType=fixdt(1, 16)  ParameterScaling=2^0  OutDataType=fixdt(1, 16)  OutScaling=2^0
  CamDownStrafe-X Proportional Gain : Gain  Gain=Cam_Down_Strafe_XPos_Kp  ParameterDataType=fixdt(1, 16)  ParameterScaling=2^0  OutDataType=fixdt(1, 16)  OutScaling=2^0
  Depth Discrete Derivative : simulink/Discrete/Discrete Derivative  SystemSampleTime=-1  gainval=1  ICPrevScaledInput=0.0  OutMin=[]  OutMax=[]  OutDataType=fixdt(1, 16)  OutScaling=2^-10  DoSatur=on
  Depth Discrete-Time Integrator : DiscreteIntegrator  gainval=1  SampleTime=-1  OutDataType=fixdt(1, 16)  OutScaling=2^0  LimitOutput=on  UpperSaturationLimit=10  LowerSaturationLimit=-10  ICPrevOutput=DiscIntNeverNeededParam  ICPrevScaledInput=DiscIntNeverNeededParam
  Gain : Gain  Gain=-1  ParameterDataType=fixdt(1, 16)  ParameterScaling=2^0  OutDataType=fixdt(1, 16)  OutScaling=2^0
  Sum : Sum  Inputs=+++  OutDataType=sfix(16)  OutScaling=2^0  SaturateOnIntegerOverflow=on  InputSameDT=on  OutDataTypeStr=Inherit: Same as first input
  u : Outport
  wires:
  CamDownStrafe-X Integral Gain/1 -> Depth Discrete-Time Integrator/1
  CamDownStrafe-X Derivative Gain/1 -> Depth Discrete Derivative/1
  Depth Discrete Derivative/1 -> Sum/2
  Sum/1 -> Gain/1
  CamDownStrafe-X Proportional Gain/1 -> Sum/1
  Depth Discrete-Time Integrator/1 -> Sum/3
  e/1 -> CamDownStrafe-X Integral Gain/1, CamDownStrafe-X Derivative Gain/1, CamDownStrafe-X Proportional Gain/1
  Gain/1 -> u/1

== system brain/StateFlow Functions/StateFlowFunctions.FollowOnePath.OnePath.AlignWithPath.GetHeadings/Hough Transform Stuff ==
  BW : Inport
  Hough Transform : viptransforms/Hough Transform  DialogController=vipDDGCreate  DialogControllerArgs=DataTag20  theta_res=pi/180  rho_res=1  out_theta_rho=on  outdtmode=double  firstCoeffMode=Binary point scaling  firstCoeffWordLength=16  firstCoeffFracLength=14  secondCoeffMode=Binary point scaling  secondCoeffWordLength=32  secondCoeffFracLength=16  outputMode=Binary point scaling  outputWordLength=16  outputFracLength=0  accumMode=Binary point scaling  accumWordLength=32  accumFracLength=20  prodOutputMode=Binary point scaling  prodOutputWordLength=32  prodOutputFracLength=20  memoryMode=Binary point scaling  memoryWordLength=32  memoryFracLength=16  roundingMode=Nearest  overflowMode=on
  IsLinePresent : Stateflow chart  TreatAsAtomicUnit=on
  Theta : Outport
  Rho : Outport  Port=2
  Votes : Outport  Port=3
  wires:
  Hough Transform/1 -> IsLinePresent/1(HoughTable)
  Hough Transform/2 -> IsLinePresent/2(ThetaValues)
  Hough Transform/3 -> IsLinePresent/3(RhoValues)
  IsLinePresent/1(Theta) -> Theta/1
  BW/1 -> Hough Transform/1
  IsLinePresent/2(Rho) -> Rho/1
  IsLinePresent/3(maxVotes) -> Votes/1

== system brain/StateFlow Functions/StateFlowFunctions.FollowOnePath.OnePath.CamDown_CenterOver_Yaw/X-Axis Control ==
  BlobX : Inport  OutDataType=fixdt(1, 16)  OutScaling=2^0
  CenterX : Inport  Port=2  OutDataType=fixdt(1, 16)  OutScaling=2^0
  Data Type Conversion : DataTypeConversion  OutDataTypeMode=int8  OutDataType=fixdt(1, 16)  OutScaling=2^0  OutDataTypeStr=int8  SaturateOnIntegerOverflow=on
  Data Type Conversion1 : DataTypeConversion  OutDataTypeMode=int8  OutDataType=fixdt(1, 16)  OutScaling=2^0  OutDataTypeStr=int8  SaturateOnIntegerOverflow=on
  Gain : Gain  Gain=-1  ParameterDataType=fixdt(1, 16)  ParameterScaling=2^0  OutDataType=fixdt(1, 16)  OutScaling=2^0
  PID Controller X Position : Subsystem  Description=PID
  Subtract : Sum  Inputs=-+  OutDataTypeMode=double  OutDataType=fixdt(1, 16)  OutScaling=2^-10  OutDataTypeStr=double
  Left1 : Outport  OutDataType=fixdt(1, 16)  OutScaling=2^0
  Right1 : Outport  Port=2  OutDataType=fixdt(1, 16)  OutScaling=2^0
  wires:
  CenterX/1 -> Subtract/1
  BlobX/1 -> Subtract/2
  Subtract/1 -> PID Controller X Position/1(e)  "Error"
  PID Controller X Position/1(u) -> Data Type Conversion/1
  Data Type Conversion/1 -> Left1/1, Gain/1
  Gain/1 -> Data Type Conversion1/1
  Data Type Conversion1/1 -> Right1/1

== system brain/StateFlow Functions/StateFlowFunctions.FollowOnePath.OnePath.CamDown_CenterOver_Yaw/Y-Axis Control ==
  BlobY : Inport  OutDataType=fixdt(1, 16)  OutScaling=2^0
  CenterY : Inport  Port=2  OutDataType=fixdt(1, 16)  OutScaling=2^0
  Data Type Conversion : DataTypeConversion  OutDataTypeMode=int8  OutDataType=fixdt(1, 16)  OutScaling=2^0  OutDataTypeStr=int8  SaturateOnIntegerOverflow=on
  PID Controller Y Axis : Subsystem  Description=PID
  Subtract : Sum  Inputs=+-  OutDataTypeMode=double  OutDataType=fixdt(1, 16)  OutScaling=2^-10  OutDataTypeStr=double
  ChangetoForward : Outport  OutDataType=fixdt(1, 16)  OutScaling=2^0
  wires:
  CenterY/1 -> Subtract/1
  BlobY/1 -> Subtract/2
  Subtract/1 -> PID Controller Y Axis/1(e)  "Error"
  PID Controller Y Axis/1(u) -> Data Type Conversion/1
  Data Type Conversion/1 -> ChangetoForward/1

== system brain/StateFlow Functions/StateFlowFunctions.FollowOnePath.OnePath.CenterOver_Strafe/X-Axis Control ==
  BlobX : Inport  OutDataType=fixdt(1, 16)  OutScaling=2^0
  CenterX : Inport  Port=2  OutDataType=fixdt(1, 16)  OutScaling=2^0
  Data Type Conversion : DataTypeConversion  OutDataTypeMode=int8  OutDataType=fixdt(1, 16)  OutScaling=2^0  OutDataTypeStr=int8  SaturateOnIntegerOverflow=on
  PID Controller X Position : Subsystem  Description=PID
  Subtract : Sum  Inputs=+-  OutDataTypeMode=double  OutDataType=fixdt(1, 16)  OutScaling=2^-10  OutDataTypeStr=double
  Strafe1 : Outport  OutDataType=fixdt(1, 16)  OutScaling=2^0
  wires:
  CenterX/1 -> Subtract/1
  BlobX/1 -> Subtract/2
  Subtract/1 -> PID Controller X Position/1(e)  "Error"
  PID Controller X Position/1(u) -> Data Type Conversion/1
  Data Type Conversion/1 -> Strafe1/1

== system brain/StateFlow Functions/StateFlowFunctions.FollowOnePath.OnePath.CenterOver_Strafe/Y-Axis Control ==
  BlobY : Inport  OutDataType=fixdt(1, 16)  OutScaling=2^0
  CenterY : Inport  Port=2  OutDataType=fixdt(1, 16)  OutScaling=2^0
  Data Type Conversion : DataTypeConversion  OutDataTypeMode=int8  OutDataType=fixdt(1, 16)  OutScaling=2^0  OutDataTypeStr=int8  SaturateOnIntegerOverflow=on
  PID Controller Y Axis : Subsystem  Description=PID
  Subtract : Sum  Inputs=+-  OutDataTypeMode=double  OutDataType=fixdt(1, 16)  OutScaling=2^-10  OutDataTypeStr=double
  ChangetoForward : Outport  OutDataType=fixdt(1, 16)  OutScaling=2^0
  wires:
  CenterY/1 -> Subtract/1
  BlobY/1 -> Subtract/2
  Subtract/1 -> PID Controller Y Axis/1(e)  "Error"
  PID Controller Y Axis/1(u) -> Data Type Conversion/1
  Data Type Conversion/1 -> ChangetoForward/1

== system brain/StateFlow Functions/StateFlowFunctions.FollowOnePath.OnePath.HSVSegmentation/Segmentation ==
  H : Inport
  S : Inport  Port=2  OutDataType=fixdt(1, 16)  OutScaling=2^0
  Data Type Conversion : DataTypeConversion  OutDataTypeMode=boolean  OutDataType=fixdt(1, 16)  OutScaling=2^0  OutDataTypeStr=boolean
  Erosion : vipmorphops/Erosion  nhoodsrc=Specify via dialog  strel=strel('square',4)
  Hue Higher Comparison : simulink/Logic and Bit Operations/Compare To Constant  SystemSampleTime=-1  relop=>  const=Track_HueHigher  LogicOutDataTypeMode=boolean  ZeroCross=off
  Hue Lower Comparison : simulink/Logic and Bit Operations/Compare To Constant  SystemSampleTime=-1  relop=<  const=Track_HueLower  LogicOutDataTypeMode=boolean  ZeroCross=off
  Logical Operator : Logic  Operator=OR  AllPortsSameDT=off  OutDataTypeMode=boolean  LogicDataType=fixdt(0, 8)  OutDataTypeStr=boolean
  Logical Operator1 : Logic  AllPortsSameDT=off  OutDataTypeMode=boolean  LogicDataType=fixdt(0, 8)  OutDataTypeStr=boolean
  Saturation Comparison : simulink/Logic and Bit Operations/Compare To Constant  SystemSampleTime=-1  relop=>  const=Track_Saturation  LogicOutDataTypeMode=boolean  ZeroCross=off
  BW : Outport
  wires:
  Data Type Conversion/1 -> BW/1
  Erosion/1 -> Data Type Conversion/1
  H/1 -> Hue Lower Comparison/1, Hue Higher Comparison/1
  Hue Lower Comparison/1 -> Logical Operator/1
  Hue Higher Comparison/1 -> Logical Operator/2
  S/1 -> Saturation Comparison/1
  Logical Operator/1 -> Logical Operator1/1
  Saturation Comparison/1 -> Logical Operator1/2
  Logical Operator1/1 -> Erosion/1  "BW"

== system brain/StateFlow Functions/StateFlowFunctions.FollowOnePath.RecognizePath.LookforTrack/LookforTrack ==
  H : Inport
  S : Inport  Port=2  OutDataType=fixdt(1, 16)  OutScaling=2^0
  Blob Analysis : vipstatistics/Blob Analysis  Tag=vipblks_row_conv  DialogController=vipDDGCreate  DialogControllerArgs=DataTag24  area=off  centroid=off  bBox=off  majorAxis=off  minorAxis=off  angle=off  eccentricity=on  equivDiameterSq=off  extent=off  perimeter=off  maxBlobs=Max_Num_Blobs  warnIfNumBlobsExceeded=on  isCount=off  useMinArea=on  minArea=Min_Blob_Size  useMaxArea=on  maxArea=Max_Blob_Size  excludeBorderBlob=off  outDT=single  isOutVarDim=off  isFill=on  fillValues=-1  conn=8  isLabel=off  outputMode=Binary point scaling  outputWordLength=32  outputFracLength=16  firstCoeffMode=Binary point scaling  firstCoeffWordLength=16  firstCoeffFracLength=14  secondCoeffMode=Binary point scaling  secondCoeffWordLength=32  secondCoeffFracLength=16  accumMode=Binary point scaling  accumWordLength=32  accumFracLength=0  prodOutputMode=Binary point scaling  prodOutputWordLength=32  prodOutputFracLength=16  roundingMode=Floor  overflowMode=off
  CheckConditions : Stateflow chart  TreatAsAtomicUnit=on
  Constant : Constant  Value=Track_Min_Eccentricity  OutDataType=fixdt(1, 16)  OutScaling=2^0  SampleTime=-1
  Hue Higher Comparison : simulink/Logic and Bit Operations/Compare To Constant  SystemSampleTime=-1  relop=>  const=Track_HueHigher  LogicOutDataTypeMode=boolean  ZeroCross=off
  Hue Lower Comparison : simulink/Logic and Bit Operations/Compare To Constant  SystemSampleTime=-1  relop=<  const=Track_HueLower  LogicOutDataTypeMode=boolean  ZeroCross=off
  Logical Operator : Logic  Operator=OR  AllPortsSameDT=off  OutDataTypeMode=boolean  LogicDataType=fixdt(0, 8)  OutDataTypeStr=boolean
  Logical Operator1 : Logic  AllPortsSameDT=off  OutDataTypeMode=boolean  LogicDataType=fixdt(0, 8)  OutDataTypeStr=boolean
  Saturation Comparison : simulink/Logic and Bit Operations/Compare To Constant  SystemSampleTime=-1  relop=>  const=Track_Saturation  LogicOutDataTypeMode=boolean  ZeroCross=off
  BWout : Outport  OutDataType=fixdt(1, 16)  OutScaling=2^0
  Image : Outport  Port=2  OutDataType=fixdt(1, 16)  OutScaling=2^0
  wires:
  H/1 -> Hue Lower Comparison/1, Hue Higher Comparison/1
  Hue Lower Comparison/1 -> Logical Operator/1
  Hue Higher Comparison/1 -> Logical Operator/2
  Blob Analysis/1 -> CheckConditions/1(Eccent)
  S/1 -> Saturation Comparison/1
  Logical Operator/1 -> Logical Operator1/1
  Saturation Comparison/1 -> Logical Operator1/2
  Logical Operator1/1 -> Blob Analysis/1, BWout/1  "BW"
  Constant/1 -> CheckConditions/2(Track_Min_Eccentricity)
  CheckConditions/1(Image) -> Image/1
